simulink model "SLIP_ratio"  (R2015a)
settings: Solver=ode45  StartTime=0.0  StopTime=10.0  RelTol=1e-3
settings Model: Creator=BML  LastModifiedBy=BML

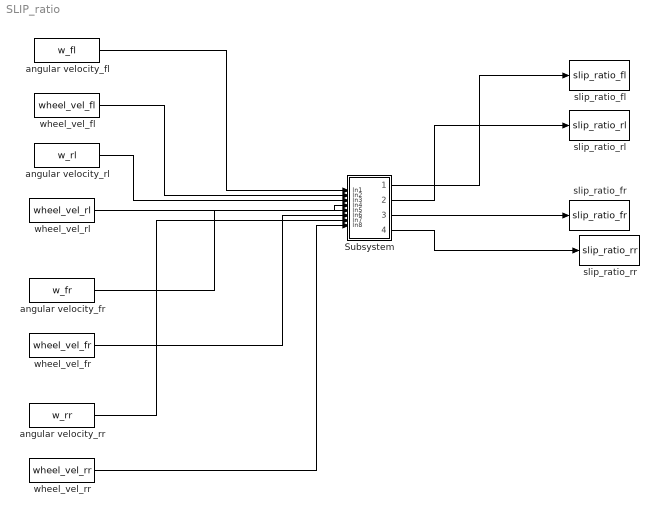
== system SLIP_ratio ==
  Subsystem : Subsystem
  angular velocity_fl : FromWorkspace  VariableName=w_fl  SampleTime=0
  angular velocity_fr : FromWorkspace  VariableName=w_fr  SampleTime=0
  angular velocity_rl : FromWorkspace  VariableName=w_rl  SampleTime=0
  angular velocity_rr : FromWorkspace  VariableName=w_rr  SampleTime=0
  slip_ratio_fl : ToWorkspace  VariableName=slip_ratio_fl  SaveFormat=Timeseries  SampleTime=-1
  slip_ratio_fr : ToWorkspace  VariableName=slip_ratio_fr  SaveFormat=Timeseries  SampleTime=-1
  slip_ratio_rl : ToWorkspace  VariableName=slip_ratio_rl  SaveFormat=Timeseries  SampleTime=-1
  slip_ratio_rr : ToWorkspace  VariableName=slip_ratio_rr  SaveFormat=Timeseries  SampleTime=-1
  wheel_vel_fl : FromWorkspace  VariableName=wheel_vel_fl  SampleTime=0
  wheel_vel_fr : FromWorkspace  VariableName=wheel_vel_fr  SampleTime=0
  wheel_vel_rl : FromWorkspace  VariableName=wheel_vel_rl  SampleTime=0
  wheel_vel_rr : FromWorkspace  VariableName=wheel_vel_rr  SampleTime=0
  wires:
  angular velocity_fl/1 -> Subsystem/1(In1)
  wheel_vel_fl/1 -> Subsystem/2(In2)
  angular velocity_rl/1 -> Subsystem/3(In3)
  wheel_vel_rl/1 -> Subsystem/4(In4)
  angular velocity_fr/1 -> Subsystem/5(In5)
  wheel_vel_fr/1 -> Subsystem/6(In6)
  angular velocity_rr/1 -> Subsystem/7(In7)
  wheel_vel_rr/1 -> Subsystem/8(In8)
  Subsystem/1(Out1) -> slip_ratio_fl/1
  Subsystem/2(Out2) -> slip_ratio_rl/1
  Subsystem/3(Out3) -> slip_ratio_fr/1
  Subsystem/4(Out4) -> slip_ratio_rr/1

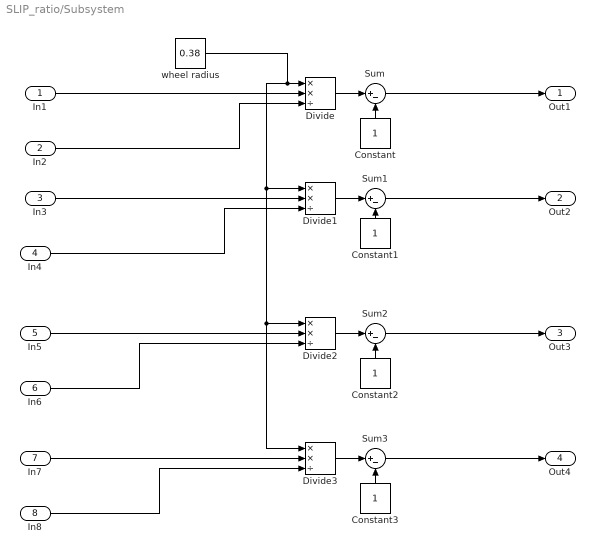
== system SLIP_ratio/Subsystem ==
  In1 : Inport
  In2 : Inport  Port=2
  In3 : Inport  Port=3
  In4 : Inport  Port=4
  In5 : Inport  Port=5
  In6 : Inport  Port=6
  In7 : Inport  Port=7
  In8 : Inport  Port=8
  Constant{,1..3} (4 alike) : Constant
  Divide{,1..3} (4 alike) : Product  Inputs=**/
  Sum{,1..3} (4 alike) : Sum  Inputs=|+-
  wheel radius : Constant  Value=0.38
  Out1 : Outport
  Out2 : Outport  Port=2
  Out3 : Outport  Port=3
  Out4 : Outport  Port=4
  wires:
  Constant/1 -> Sum/2
  In1/1 -> Divide/2
  Sum/1 -> Out1/1
  Divide1/1 -> Sum1/1
  Constant1/1 -> Sum1/2
  In3/1 -> Divide1/2
  In2/1 -> Divide/3
  Divide/1 -> Sum/1
  In4/1 -> Divide1/3
  Constant3/1 -> Sum3/2
  In6/1 -> Divide2/3
  In7/1 -> Divide3/2
  In5/1 -> Divide2/2
  In8/1 -> Divide3/3
  Sum1/1 -> Out2/1
  Divide2/1 -> Sum2/1
  Sum2/1 -> Out3/1
  Divide3/1 -> Sum3/1
  Sum3/1 -> Out4/1
  Constant2/1 -> Sum2/2
  wheel radius/1 -> Divide3/1, Divide2/1, Divide1/1, Divide/1
